simulink model "mR52_MultiCPUSend"  (R2024a)
settings: Solver=FixedStepAuto  StartTime=0.0  StopTime=10.0  FixedStep=0.2  RelTol=1e-3  EnableMultiTasking=on
PreLoadFcn:
  | % NXP_MBDT_S32ZE callback: DO NOT REMOVE
  | mbd_s32ze.common.nxp.model_callbacks.preLoadFcn();
PostLoadFcn:
  | % NXP_MBDT_S32ZE callback: DO NOT REMOVE
  | mbd_s32ze.common.nxp.model_callbacks.postLoadFcn();
InitFcn:
  | % NXP_MBDT_S32ZE callback: DO NOT REMOVE
  | mbd_s32ze.common.nxp.model_callbacks.initFcn();
settings Model: DataDictionary=mR52_MultiCPUSend.sldd  Creator=scaliska  LastModifiedBy=nxf63265
settings SolverCC: AlgebraicLoopSolver=TrustRegion
settings DataIOCC: LimitDataPoints=on  ReturnWorkspaceOutputs=off
settings OptimizationCC: EnhancedBackFolding=on  PassReuseOutputArgsAs=Individual arguments  ZeroExternalMemoryAtStartup=off  ZeroInternalMemoryAtStartup=off  MaxStackSize=64  OptimizeBlockOrder=speed  DifferentSizesBufferReuse=on  OptimizationCustomize=off  EfficientTunableParamExpr=on
settings DebuggingCC: ParameterTunabilityLossMsg=error  UnconnectedInputMsg=warning  UnconnectedOutputMsg=warning  UnconnectedLineMsg=warning  AllowSymbolicDim=off  SFUnexpectedBacktrackingDiag=warning  SFNoUnconditionalDefaultTransitionDiag=warning  SFExecutionAtInitializationDiag=none  ArithmeticOperatorsInVariantConditions=warning
settings HardwareCC: ProdBitPerPointer=32  ProdBitPerSizeT=32  ProdBitPerPtrDiffT=32  ProdLargestAtomicInteger=Long  ProdLargestAtomicFloat=Double  ProdWordSize=32  ProdHWDeviceType=ARM Compatible->ARM Cortex
settings ModelReferenceCC: EnableRefExpFcnMdlSchedulingChecks=on  ModelReferenceNumInstancesAllowed=Single  PropagateSignalLabelsOutOfModel=off
settings SFSimCC: SimUseLocalCustomCode=off  MATLABDynamicMemAlloc=off  CustomCodeUndefinedFunction=UseInterfaceOnly
settings RTWCC: Description=Embedded Coder  SystemTargetFile=ert.tlc  HardwareBoard=NXP S32ZE2xx  TemplateMakefile=ert_default_tmf  RTWUseLocalCustomCode=off  Toolchain=NXP S32 Design Studio GCC (S32ZE)  GPUComputeCapability=3.5
settings CodeAppCC: ForceParamTrailComments=on  IgnoreCustomStorageClasses=off  MaxIdLength=63  OperatorAnnotations=on  SimulinkDataObjDesc=on  SFDataObjDesc=on  InsertBlockDesc=on
settings ERTTargetCC: SupportContinuousTime=on  ERTSrcFileBannerTemplate=mbd_s32ze_ert_code_template.cgt  ERTHdrFileBannerTemplate=mbd_s32ze_ert_code_template.cgt  ERTDataSrcFileTemplate=mbd_s32ze_ert_code_template.cgt  ERTDataHdrFileTemplate=mbd_s32ze_ert_code_template.cgt
settings ConfigComp: CovMetricSettings=dw  CovSaveCumulativeToWorkspaceVar=on  CovSaveSingleToWorkspaceVar=on  CovExternalEMLEnable=off

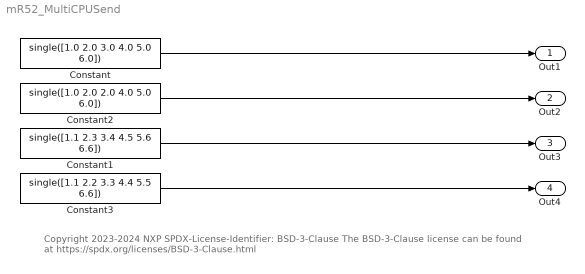
== system mR52_MultiCPUSend ==
  note: Copyright 2023-2024 NXP
      |
      | SPDX-License-Identifier: BSD-3-Clause
      | The BSD-3-Clause license can be found at https://spdx.org/licenses/BSD-3-Clause.html
  Constant : Constant  Value=single([1.0 2.0 3.0 4.0 5.0 6.0])  SampleTime=0
  Constant1 : Constant  Value=single([1.1 2.3 3.4 4.5 5.6 6.6])  SampleTime=0
  Constant2 : Constant  Value=single([1.0 2.0 2.0 4.0 5.0 6.0])  SampleTime=0
  Constant3 : Constant  Value=single([1.1 2.2 3.3 4.4 5.5 6.6])  SampleTime=0
  Out1 : Outport  OutDataTypeStr=single  PortDimensions=[1 6]
  Out2 : Outport  Port=2  OutDataTypeStr=single  PortDimensions=[1 6]
  Out3 : Outport  Port=3  OutDataTypeStr=single  PortDimensions=[1 6]
  Out4 : Outport  Port=4  OutDataTypeStr=single  PortDimensions=[1 6]
  wires:
  Constant/1 -> Out1/1
  Constant1/1 -> Out3/1
  Constant2/1 -> Out2/1
  Constant3/1 -> Out4/1
